simulink model "noise"  (R2017a)
settings: Solver=VariableStepAuto  StartTime=0.0  StopTime=10  RelTol=1e-3
values from neighbouring files (symbols this model uses):
  Ts = 1/(15)    (= 0.0666666666667)    [Inv.m]
undefined symbols (not defined in the file or in its folder): A, B, C, D
libraries: simulink x1
settings Model: Creator=cl38301  LastModifiedBy=cl38301

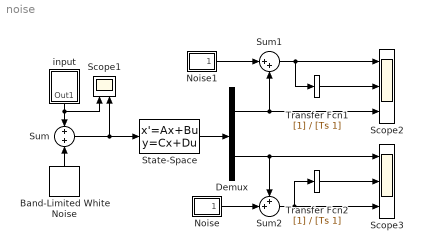
== system noise ==
  Band-Limited White Noise : simulink/Sources/Band-Limited White Noise  Cov=[0.01]  Ts=0.1  seed=[23341]
  Demux : Demux  Outputs=2
  Noise : Subsystem
  Noise1 : Subsystem
  Scope1 : Scope  NumInputPorts=2
  Scope2 : Scope  NumInputPorts=3
  Scope3 : Scope  NumInputPorts=3
  State-Space : StateSpace  A=A  B=B  C=C  D=D  X0=0
  Sum : Sum
  Sum1 : Sum  Inputs=|++
  Sum2 : Sum  Inputs=++|
  Transfer Fcn1 : TransferFcn  Denominator=[Ts 1]
  Transfer Fcn2 : TransferFcn  Denominator=[Ts 1]
  input : Subsystem
  wires:
  State-Space/1 -> Demux/1
  input/1(Out1) -> Sum/1, Scope1/1
  Band-Limited White Noise/1 -> Sum/2
  Sum/1 -> State-Space/1, Scope1/2
  Demux/2 -> Scope3/1, Sum2/1
  Sum2/1 -> Scope3/3, Transfer Fcn2/1
  Demux/1 -> Sum1/2, Scope2/3
  Sum1/1 -> Transfer Fcn1/1, Scope2/1
  Noise1/1(Out1) -> Sum1/1
  Transfer Fcn1/1 -> Scope2/2
  Noise/1(Out1) -> Sum2/2
  Transfer Fcn2/1 -> Scope3/2

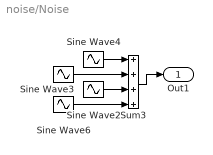
== system noise/Noise ==
  Sine Wave2 : Sin  Amplitude=0.06  Frequency=76  SampleTime=0
  Sine Wave3 : Sin  Amplitude=0.01  Frequency=79  SampleTime=0
  Sine Wave4 : Sin  Amplitude=0.02  Frequency=102  SampleTime=0
  Sine Wave6 : Sin  Amplitude=0.04  Frequency=123  SampleTime=0
  Sum3 : Sum  Inputs=++++
  Out1 : Outport
  wires:
  Sine Wave3/1 -> Sum3/2
  Sine Wave2/1 -> Sum3/3
  Sum3/1 -> Out1/1
  Sine Wave4/1 -> Sum3/1
  Sine Wave6/1 -> Sum3/4

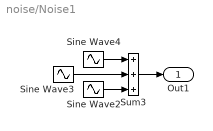
== system noise/Noise1 ==
  Sine Wave2 : Sin  Amplitude=0.06  Frequency=80  SampleTime=0
  Sine Wave3 : Sin  Amplitude=0.01  Frequency=54  SampleTime=0
  Sine Wave4 : Sin  Amplitude=0.02  Frequency=150  SampleTime=0
  Sum3 : Sum  Inputs=+++
  Out1 : Outport
  wires:
  Sine Wave3/1 -> Sum3/2
  Sine Wave2/1 -> Sum3/3
  Sum3/1 -> Out1/1
  Sine Wave4/1 -> Sum3/1

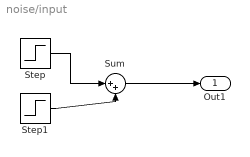
== system noise/input ==
  Step : Step  After=2  SampleTime=0
  Step1 : Step  Time=3  After=-2  SampleTime=0
  Sum : Sum  Inputs=|++
  Out1 : Outport
  wires:
  Step/1 -> Sum/1
  Sum/1 -> Out1/1
  Step1/1 -> Sum/2
